simulink model "hcu_main_ADASwEPS"  (Simulink 8.2)
settings: Solver=FixedStepDiscrete  StartTime=0.0  StopTime=inf  FixedStep=0.001  RelTol=1e-3
PostLoadFcn:
  | , if any(exist('dsrtsu_mdlpostloadfcn', 'file') == [2, 3, 6]), try dsrtsu_mdlpostloadfcn('Execute', bdroot); catch fprintf('Error in PostLoadFcn (dsrtsu_mdlpostloadfcn) for model "%s":\n %s\n', bdroot, lasterr); end, end,
values from neighbouring files (symbols this model uses):
  C_TASK_1MS_S = (	C_TICK_TIME_S       )    [hcu_local_hdr.m]    (also in temp_ovrd_values.m = double(	0.001                  ))
  C_TICK_TIME_S = single(	0.005	    	)    [hcu_local_hdr.m]
  ENUM_EPSLFCSTATUS_ACTIVE = uint8(  2  )    [hcu_local_hdr.m]
  ENUM_EPSLFCSTATUS_TRANSITION = uint8(  3  )    [hcu_local_hdr.m]
  ENUM_EPSLKASTATUS_ACTIVE = uint8(  2  )    [hcu_local_hdr.m]
  ENUM_EPSMODEREQ_ANGLE = uint8(  1  )    [hcu_local_hdr.m]
  ENUM_EPSMODEREQ_INTERNAL = uint8(  0  )    [hcu_local_hdr.m]
  ENUM_EPSMODEREQ_TORQUE = uint8(  2  )    [hcu_local_hdr.m]
  ENUM_GEARPOSN_1ST = uint8(  1  )    [hcu_local_hdr.m]
  ENUM_GEARPOSN_2ND = uint8(  2  )    [hcu_local_hdr.m]
  ENUM_GEARPOSN_3RD = uint8(  3  )    [hcu_local_hdr.m]
  ENUM_GEARPOSN_4TH = uint8(  4  )    [hcu_local_hdr.m]
  ENUM_GEARPOSN_5TH = uint8(  5  )    [hcu_local_hdr.m]
  ENUM_GEARPOSN_6TH = uint8(  6  )    [hcu_local_hdr.m]
  ENUM_GEARPOSN_R = uint8(  7  )    [hcu_local_hdr.m]
  FALSE = boolean( 0 )    [hcu_local_hdr.m]
  TRUE = boolean( 1 )    [hcu_local_hdr.m]
undefined symbols (not defined in the file or in its folder): AISP_EPSCurrent_pct, AISP_TqASensorDelta_pct, AISP_TqBSensorDelta_pct, dHAL_IN, hal, INVALID_ABS1_TIMEOUT, INVALID_ABS2_TIMEOUT, INVALID_ABS3_TIMEOUT, INVALID_ABS4_TIMEOUT, INVALID_AC1_TIMEOUT, INVALID_ADASTORQ_REQ, INVALID_BCM1_TIMEOUT, INVALID_BCM2_TIMEOUT, INVALID_BOOSTER_VAC, INVALID_CSW1_TIMEOUT, INVALID_CUR_VEHDECE, INVALID_CURBRAKEDECE_REQ, INVALID_CURSTEERANG_REQ, INVALID_CURSTEERTQ_REQ, INVALID_ECM1_TIMEOUT, INVALID_ECM2_TIMEOUT, INVALID_ECM3_TIMEOUT, INVALID_ECM9_TIMEOUT, INVALID_ENG_TORQUE_FRICTIONAL, INVALID_ENG_TORQUE_INDICATED, INVALID_ENG_TORQUE_INDICATEDCOR, INVALID_ENG_TQ_MAX, INVALID_ENG_TQ_MIN, INVALID_EPAS2_TIMEOUT, INVALID_EPAS3_TIMEOUT, INVALID_EPB1_TIMEOUT, INVALID_EPS_BATTVOLT, INVALID_ESC_BATTVOLT, INVALID_GRADE, INVALID_HCU3_TIMEOUT, INVALID_HCU4_TIMEOUT, INVALID_HMI1_TIMEOUT, INVALID_HMI2_TIMEOUT, INVALID_LAT_ACC, INVALID_LONG_ACC, INVALID_MC_PRESSURE, INVALID_METER1_TIMEOUT, INVALID_METER3_TIMEOUT, INVALID_METER_VEHSPD, INVALID_ODO_METER, INVALID_OUTSIDE_TEMP, INVALID_PARKBRAKEBIND_STAT, INVALID_PEDALTQ_REQ, INVALID_SAS1_TIMEOUT, INVALID_SAS_ANGLE, INVALID_SHIFTER_POSN, INVALID_TCM1_TIMEOUT, INVALID_TCM2_TIMEOUT, INVALID_VCU1_TIMEOUT, INVALID_VCU2_TIMEOUT, INVALID_VEH_CRASH, INVALID_VEH_SPD, INVALID_WHEEL_SPD, INVALID_YAW_RATE, KHAL_MssgIdObj1_num ... (+8)
libraries: simulink x147, hcu_lib x38, rti1401lib_dio_type3 x4, rtimmsu_dsrtlib x3, app x1, rtiethernetudplib x1, rti1401lib_adc_type4 x1, rti1401lib_dac_type3 x1, inp x1, lidr x1, outp x1
(part 12 of 15)

== system hcu_main_ADASwEPS/dHAL_IN/HAL_IN_HMI/BO__1347_HMI1__8_HMI ==
  CAN1_Rx : Inport
  Bus Selector : BusSelector  OutputSignals=HMI1.ACCCancel,HMI1.ACCOn,HMI1.ACCRes_SpdInc,HMI1.ACCSet_SpdDec,HMI1.ACCSpeedDec,HMI1.ACCSpeedInc,HMI1.ACCTimeGapDec,HMI1.ACCTimeGapInc,HMI1.AEBEnable,HMI1.CSCEnable,HMI1.FCWEnable,HMI1.IGSAOn,HMI1.IGSARes_SpdInc,HMI1.IGSASet_SpdDec,HMI1.IGSASwitchMode,HMI1.LCSEnable,HMI1.LFC_PilotCancel,HMI1.LFC_PilotOn,HMI1.LKAEnable,HMI1.MAPAEnable,HMI1.FCWWarningMode,HMI1.DefMaxACCSetSpeed
  ACCCancel : Outport
  ACCOn : Outport  Port=2
  ACCRes_SpdInc : Outport  Port=3
  ACCSet_SpdDec : Outport  Port=4
  ACCSpeedDec : Outport  Port=5
  ACCSpeedInc : Outport  Port=6
  ACCTimeGapDec : Outport  Port=7
  ACCTimeGapInc : Outport  Port=8
  AEBEnable : Outport  Port=9
  CSCEnable : Outport  Port=10
  FCWEnable : Outport  Port=11
  IGSAOn : Outport  Port=12
  IGSARes_SpdInc : Outport  Port=13
  IGSASet_SpdDec : Outport  Port=14
  IGSASwitchMode : Outport  Port=15
  LCSEnable : Outport  Port=16
  LFC_PilotCancel : Outport  Port=17
  LFC_PilotOn : Outport  Port=18
  LKAEnable : Outport  Port=19
  MAPAEnable : Outport  Port=20
  FCWWarningMode : Outport  Port=21
  DefMaxACCSetSpeed : Outport  Port=22
  wires:
  [CAN1_Rx] -> Bus Selector/1
  CAN1_Rx/1 -> [CAN1_Rx]
  Bus Selector/1 -> ACCCancel/1  "<ACCCancel>"
  Bus Selector/2 -> ACCOn/1  "<ACCOn>"
  Bus Selector/3 -> ACCRes_SpdInc/1  "<ACCRes_SpdInc>"
  Bus Selector/4 -> ACCSet_SpdDec/1  "<ACCSet_SpdDec>"
  Bus Selector/5 -> ACCSpeedDec/1  "<ACCSpeedDec>"
  Bus Selector/6 -> ACCSpeedInc/1  "<ACCSpeedInc>"
  Bus Selector/7 -> ACCTimeGapDec/1  "<ACCTimeGapDec>"
  Bus Selector/8 -> ACCTimeGapInc/1  "<ACCTimeGapInc>"
  Bus Selector/9 -> AEBEnable/1  "<AEBEnable>"
  Bus Selector/10 -> CSCEnable/1  "<CSCEnable>"
  Bus Selector/11 -> FCWEnable/1  "<FCWEnable>"
  Bus Selector/16 -> LCSEnable/1  "<LCSEnable>"
  Bus Selector/17 -> LFC_PilotCancel/1  "<LFC_PilotCancel>"
  Bus Selector/18 -> LFC_PilotOn/1  "<LFC_PilotOn>"
  Bus Selector/19 -> LKAEnable/1  "<LKAEnable>"
  Bus Selector/20 -> MAPAEnable/1  "<MAPAEnable>"
  Bus Selector/12 -> IGSAOn/1  "<IGSAOn>"
  Bus Selector/13 -> IGSARes_SpdInc/1  "<IGSARes_SpdInc>"
  Bus Selector/14 -> IGSASet_SpdDec/1  "<IGSASet_SpdDec>"
  Bus Selector/15 -> IGSASwitchMode/1  "<IGSASwitchMode>"
  Bus Selector/21 -> FCWWarningMode/1  "<FCWWarningMode>"
  Bus Selector/22 -> DefMaxACCSetSpeed/1  "<DefMaxACCSetSpeed>"

== system hcu_main_ADASwEPS/dHAL_IN/HAL_IN_RadObjDecoder/RObj_Parser ==
  RObj_Status : Inport
  RObj_Frames1 : Inport  Port=2
  RObj_Frames2 : Inport  Port=3
  RObj_CollDetWarn : Inport  Port=4
  Ground : Ground
  Ground1 : Ground
  RObj_FramesParser : MATLAB Function  TreatAsAtomicUnit=on
  RObj_StatusParser : MATLAB Function  TreatAsAtomicUnit=on
  Terminator : Terminator
  VHAL_RadNofObjects_num : Outport
  VHAL_MeasCounter_num : Outport  Port=2
  VHAL_SensorRxInvalid_enum : Outport  Port=3
  VHAL_SensorSupplyVoltage_V : Outport  Port=4
  VHAL_SensorDefective_enum : Outport  Port=5
  VHAL_SensorMisaligned_enum : Outport  Port=6
  VHAL_SensorSwitchedOff_enum : Outport  Port=7
  VHAL_SensorExternalDisturbed_enum : Outport  Port=8
  VHAL_SensorOutputReduced_enum : Outport  Port=9
  VHAL_LatDistToborderLeft_m : Outport  Port=10
  VHAL_LatDistToborderRight_m : Outport  Port=11
  VHAL_RadObjRolCountVect40_num : Outport  Port=12
  VHAL_RadObjIDVect40_num : Outport  Port=13
  VHAL_RadObjXDisplVect40_m : Outport  Port=14
  VHAL_RadObjVrelXVect40_mps : Outport  Port=15
  VHAL_RadObjAccelXVect40_mps2 : Outport  Port=16
  VHAL_RadObjYDisplVect40_m : Outport  Port=17
  VHAL_RadObjDynPropVect40_enum : Outport  Port=18
  VHAL_RadObjPExistVect40_enum : Outport  Port=19
  VHAL_RadObjMeasStatVect40_enum : Outport  Port=20
  VHAL_RadObjWidthVect40_m : Outport  Port=21
  VHAL_RadObjLengthVect40_m : Outport  Port=22
  VHAL_RadObjRCSVect40_num : Outport  Port=23
  VHAL_RadObjVrelYVect40_mps : Outport  Port=24
  VHAL_RadObjProbVect40_num : Outport  Port=25
  VHAL_RadWarningLevel_enum : Outport  Port=26
  VHAL_RadWarningObjID_num : Outport  Port=27
  wires:
  RObj_Status/1 -> RObj_StatusParser/1(Status_Frame)
  RObj_FramesParser/1(Obj_RolCount) -> VHAL_RadObjRolCountVect40_num/1
  RObj_FramesParser/2(Obj_ID) -> VHAL_RadObjIDVect40_num/1
  RObj_FramesParser/3(Obj_LongDispl) -> VHAL_RadObjXDisplVect40_m/1
  RObj_FramesParser/4(Obj_VrelLong) -> VHAL_RadObjVrelXVect40_mps/1
  RObj_FramesParser/5(Obj_AccelLong) -> VHAL_RadObjAccelXVect40_mps2/1
  RObj_FramesParser/6(Obj_LatDispl) -> VHAL_RadObjYDisplVect40_m/1
  RObj_FramesParser/7(Obj_DynProp) -> VHAL_RadObjDynPropVect40_enum/1
  RObj_FramesParser/9(Obj_MeasStat) -> VHAL_RadObjMeasStatVect40_enum/1
  RObj_FramesParser/11(Obj_Length) -> VHAL_RadObjLengthVect40_m/1
  RObj_FramesParser/8(Obj_ProbOfExist) -> VHAL_RadObjPExistVect40_enum/1
  RObj_FramesParser/10(Obj_Width) -> VHAL_RadObjWidthVect40_m/1
  RObj_FramesParser/14(Obj_ObstacleProb) -> VHAL_RadObjProbVect40_num/1
  RObj_FramesParser/12(Obj_RCSValue) -> VHAL_RadObjRCSVect40_num/1
  RObj_FramesParser/13(Obj_LatSpeed) -> VHAL_RadObjVrelYVect40_mps/1
  RObj_Frames1/1 -> RObj_FramesParser/1(Frames1)
  RObj_Frames2/1 -> RObj_FramesParser/2(Frames2)
  RObj_StatusParser/1(N_of_Objects) -> VHAL_RadNofObjects_num/1
  RObj_StatusParser/6(SensorMisaligned) -> VHAL_SensorMisaligned_enum/1
  RObj_StatusParser/5(SensorDefective) -> VHAL_SensorDefective_enum/1
  RObj_StatusParser/8(SensorExternalDisturbed) -> VHAL_SensorExternalDisturbed_enum/1
  RObj_StatusParser/7(SensorSwitchedOff) -> VHAL_SensorSwitchedOff_enum/1
  RObj_StatusParser/9(SensorOutputReduced) -> VHAL_SensorOutputReduced_enum/1
  RObj_StatusParser/11(LatDistToborderRight) -> VHAL_LatDistToborderRight_m/1
  RObj_StatusParser/2(MeasCounter) -> VHAL_MeasCounter_num/1
  RObj_StatusParser/10(LatDistToborderLeft) -> VHAL_LatDistToborderLeft_m/1
  RObj_StatusParser/3(SensorRxInvalid) -> VHAL_SensorRxInvalid_enum/1
  RObj_StatusParser/4(SensorSupplyVoltage) -> VHAL_SensorSupplyVoltage_V/1
  RObj_CollDetWarn/1 -> Terminator/1
  Ground/1 -> VHAL_RadWarningLevel_enum/1
  Ground1/1 -> VHAL_RadWarningObjID_num/1

== system hcu_main_ADASwEPS/dHAL_IN/HAL_IN_RadObjDecoder/RObjectPackFrame ==
  CAN_Frames : Inport
  CaptureMessage1 : Inport  Port=2
  CaptureMessage2 : Inport  Port=3
  CaptureMessage3 : Inport  Port=4
  CaptureMessage4 : Inport  Port=5
  CaptureMessage5 : Inport  Port=6
  CaptureMessage6 : Inport  Port=7
  CaptureMessage7 : Inport  Port=8
  CaptureMessage8 : Inport  Port=9
  CaptureMessage9 : Inport  Port=10
  CaptureMessage10 : Inport  Port=11
  CaptureMessage11 : Inport  Port=12
  CaptureMessage12 : Inport  Port=13
  CaptureMessage13 : Inport  Port=14
  CaptureMessage14 : Inport  Port=15
  CaptureMessage15 : Inport  Port=16
  CaptureMessage16 : Inport  Port=17
  CaptureMessage17 : Inport  Port=18
  CaptureMessage18 : Inport  Port=19
  CaptureMessage19 : Inport  Port=20
  CaptureMessage20 : Inport  Port=21
  CaptureMessage21 : Inport  Port=22
  CaptureMessage22 : Inport  Port=23
  CaptureMessage23 : Inport  Port=24
  CaptureMessage24 : Inport  Port=25
  CaptureMessage25 : Inport  Port=26
  Bus Selector5 : BusSelector  OutputSignals=Status,ID,RAW_Byte_1,RAW_Byte_2,RAW_Byte_3,RAW_Byte_4,RAW_Byte_5,RAW_Byte_6,RAW_Byte_7,RAW_Byte_8
  Delay : Delay  DelayLength=1  InitialCondition=0
  For Iterator : ForIterator  IterationSource=external  IterationLimit=25
  Multiport Switch : MultiPortSwitch  Inputs=25
  RObjects_Decoder_v2 : Subsystem
  R_Objects_out : Outport  OutDataTypeStr=Bus: R_Objects
  wires:
  CaptureMessage1/1 -> Multiport Switch/2
  For Iterator/1 -> Multiport Switch/1
  CaptureMessage2/1 -> Multiport Switch/3
  CaptureMessage3/1 -> Multiport Switch/4
  CaptureMessage4/1 -> Multiport Switch/5
  CaptureMessage5/1 -> Multiport Switch/6
  CaptureMessage6/1 -> Multiport Switch/7
  CaptureMessage7/1 -> Multiport Switch/8
  CaptureMessage8/1 -> Multiport Switch/9
  CaptureMessage9/1 -> Multiport Switch/10
  CaptureMessage10/1 -> Multiport Switch/11
  CaptureMessage11/1 -> Multiport Switch/12
  CaptureMessage12/1 -> Multiport Switch/13
  CaptureMessage13/1 -> Multiport Switch/14
  CaptureMessage14/1 -> Multiport Switch/15
  CaptureMessage15/1 -> Multiport Switch/16
  CaptureMessage16/1 -> Multiport Switch/17
  CaptureMessage17/1 -> Multiport Switch/18
  CaptureMessage18/1 -> Multiport Switch/19
  CaptureMessage19/1 -> Multiport Switch/20
  CaptureMessage20/1 -> Multiport Switch/21
  CaptureMessage21/1 -> Multiport Switch/22
  CaptureMessage22/1 -> Multiport Switch/23
  CaptureMessage23/1 -> Multiport Switch/24
  CaptureMessage24/1 -> Multiport Switch/25
  CaptureMessage25/1 -> Multiport Switch/26
  RObjects_Decoder_v2/1(R_Objects_out) -> Delay/1, R_Objects_out/1
  Multiport Switch/1 -> Bus Selector5/1
  Bus Selector5/2 -> RObjects_Decoder_v2/2(ID)  "<ID>"
  Bus Selector5/4 -> RObjects_Decoder_v2/4(Byte2)  "<RAW_Byte_2>"
  Bus Selector5/3 -> RObjects_Decoder_v2/3(Byte1)  "<RAW_Byte_1>"
  Bus Selector5/10 -> RObjects_Decoder_v2/10(Byte8)  "<RAW_Byte_8>"
  Bus Selector5/1 -> RObjects_Decoder_v2/1(Status)  "<Status>"
  Bus Selector5/8 -> RObjects_Decoder_v2/8(Byte6)  "<RAW_Byte_6>"
  Bus Selector5/9 -> RObjects_Decoder_v2/9(Byte7)  "<RAW_Byte_7>"
  Bus Selector5/5 -> RObjects_Decoder_v2/5(Byte3)  "<RAW_Byte_3>"
  Bus Selector5/7 -> RObjects_Decoder_v2/7(Byte5)  "<RAW_Byte_5>"
  Bus Selector5/6 -> RObjects_Decoder_v2/6(Byte4)  "<RAW_Byte_4>"
  Delay/1 -> RObjects_Decoder_v2/11(R_Objects_in)
  CAN_Frames/1 -> For Iterator/1

== system hcu_main_ADASwEPS/dHAL_IN/HAL_IN_VCU/ADASTqReq_cvt ==
  value : Inport
  Add : Sum  Inputs=+-
  Data Type Conversion : DataTypeConversion  OutDataTypeStr=uint32  RndMeth=Nearest
  Divide : Product  Inputs=*/
  gain : Constant  Value=single(gain)  OutDataTypeStr=single
  offset : Constant  Value=single(offset)  OutDataTypeStr=single
  raw32 : Outport
  wires:
  Data Type Conversion/1 -> raw32/1
  gain/1 -> Divide/2
  Add/1 -> Divide/1
  Divide/1 -> Data Type Conversion/1
  offset/1 -> Add/2
  value/1 -> Add/1

== system hcu_main_ADASwEPS/dHAL_IN/HAL_IN_VCU/BO__1344_HMI2__8_VCU ==
  CAN1_Rx : Inport
  Bus Selector : BusSelector  OutputSignals=HMI2.ACCOn_VCU,HMI2.ACCRes_SpdInc_VCU,HMI2.ACCSet_SpdDec_VCU,HMI2.ACCTimeGapInc_VCU,HMI2.ACCTimeGapDec_VCU,HMI2.LFCOn_VCU,HMI2.MSAOn_VCU
  ACCOn_VCU : Outport
  ACCRes_SpdInc_VCU : Outport  Port=2
  ACCSet_SpdDec_VCU : Outport  Port=3
  ACCTimeGapInc_VCU : Outport  Port=4
  ACCTimeGapDec_VCU : Outport  Port=5
  LFCOn_VCU : Outport  Port=6
  MSAOn_VCU : Outport  Port=7
  wires:
  CAN1_Rx/1 -> [CAN1_Rx]
  [CAN1_Rx] -> Bus Selector/1
  Bus Selector/1 -> ACCOn_VCU/1  "<ACCOn_VCU>"
  Bus Selector/2 -> ACCRes_SpdInc_VCU/1  "<ACCRes_SpdInc_VCU>"
  Bus Selector/3 -> ACCSet_SpdDec_VCU/1  "<ACCSet_SpdDec_VCU>"
  Bus Selector/4 -> ACCTimeGapInc_VCU/1  "<ACCTimeGapInc_VCU>"
  Bus Selector/5 -> ACCTimeGapDec_VCU/1  "<ACCTimeGapDec_VCU>"
  Bus Selector/6 -> LFCOn_VCU/1  "<LFCOn_VCU>"
  Bus Selector/7 -> MSAOn_VCU/1  "<MSAOn_VCU>"

== system hcu_main_ADASwEPS/dHAL_IN/HAL_IN_VCU/BO__1360_VCU1__8_VCU ==
  CAN1_Rx : Inport
  Bus Selector : BusSelector  OutputSignals=VCU1.CurBrakeDecReq,VCU1.CurBrakeDecReq_A,VCU1.ADASTqReq,VCU1.ADASTqReq_A,VCU1.CurVehDec,VCU1.DecContMan,VCU1.DriverBrakeSw,VCU1.DriverBrakeSw_V,VCU1.ExtTqAvail,VCU1.ECMTqSrc,VCU1.ESCBrkSta,VCU1.ESCExtBrkAvail,VCU1.VCUFault,VCU1.VCUBattVolt,VCU1.VCU1_Checksum,VCU1.VCU1_LifeCount
  ChecksumCalculation : Subsystem  TreatAsAtomicUnit=on
  CurBrakeDecReq : Outport
  CurBrakeDecReq_A : Outport  Port=2
  ADASTqReq : Outport  Port=3
  ADASTqReq_A : Outport  Port=4
  CurVehDec : Outport  Port=5
  DecContMan : Outport  Port=6
  DriverBrakeSw : Outport  Port=7
  DriverBrakeSw_V : Outport  Port=8
  ExtTqAvail : Outport  Port=9
  ECMTqSrc : Outport  Port=10
  ESCBrkSta : Outport  Port=11
  ESCExtBrkAvail : Outport  Port=12
  VCUFault : Outport  Port=13
  VCUBattVolt : Outport  Port=14
  VCU1_LifeCount : Outport  Port=15
  VCU1_Checksum : Outport  Port=16
  Message_Checksum : Outport  Port=17
  wires:
  [CAN1_Rx] -> Bus Selector/1
  CAN1_Rx/1 -> [CAN1_Rx]
  Bus Selector/1 -> CurBrakeDecReq/1  "<CurBrakeDecReq>"
  Bus Selector/5 -> CurVehDec/1  "<CurVehDec>"
  Bus Selector/6 -> DecContMan/1  "<DecContMan>"
  Bus Selector/7 -> DriverBrakeSw/1  "<DriverBrakeSw>"
  Bus Selector/2 -> CurBrakeDecReq_A/1  "<CurBrakeDecReq_A>"
  [CAN1_Rx] -> ChecksumCalculation/1(CAN1_Rx)
  ChecksumCalculation/1(Message_Checksum) -> Message_Checksum/1
  Bus Selector/3 -> ADASTqReq/1  "<ADASTqReq>"
  Bus Selector/4 -> ADASTqReq_A/1  "<ADASTqReq_A>"
  Bus Selector/8 -> DriverBrakeSw_V/1  "<DriverBrakeSw_V>"
  Bus Selector/9 -> ExtTqAvail/1  "<ExtTqAvail>"
  Bus Selector/10 -> ECMTqSrc/1  "<ECMTqSrc>"
  Bus Selector/11 -> ESCBrkSta/1  "<ESCBrkSta>"
  Bus Selector/12 -> ESCExtBrkAvail/1  "<ESCExtBrkAvail>"
  Bus Selector/13 -> VCUFault/1  "<VCUFault>"
  Bus Selector/14 -> VCUBattVolt/1  "<VCUBattVolt>"
  Bus Selector/15 -> VCU1_Checksum/1  "<VCU1_Checksum>"
  Bus Selector/16 -> VCU1_LifeCount/1  "<VCU1_LifeCount>"

== system hcu_main_ADASwEPS/dHAL_IN/HAL_IN_VCU/BO__1361_VCU2__8_VCU ==
  CAN1_Rx : Inport
  Bus Selector : BusSelector  OutputSignals=VCU2.VCU_AccelPedalPosn,VCU2.VCU_AccelPedalPosn_V,VCU2.PedalTqReq,VCU2.ADAS_GearPosnReq_ALLOW,VCU2.MSAStatus,VCU2.VCU2_LifeCount,VCU2.VCU2_Checksum
  ChecksumCalculation : Subsystem  TreatAsAtomicUnit=on
  VCU_AccelPedalPosn : Outport
  VCU_AccelPedalPosn_V : Outport  Port=2
  PedalTqReq : Outport  Port=3
  ADAS_GearPosnReq_ALLOW : Outport  Port=4
  MSAStatus : Outport  Port=5
  VCU2_LifeCount : Outport  Port=6
  VCU2_Checksum : Outport  Port=7
  Message_Checksum : Outport  Port=8
  wires:
  CAN1_Rx/1 -> [CAN1_Rx]
  [CAN1_Rx] -> Bus Selector/1
  [CAN1_Rx] -> ChecksumCalculation/1(CAN1_Rx)
  ChecksumCalculation/1(Message_Checksum) -> Message_Checksum/1
  Bus Selector/1 -> VCU_AccelPedalPosn/1  "<VCU_AccelPedalPosn>"
  Bus Selector/2 -> VCU_AccelPedalPosn_V/1  "<VCU_AccelPedalPosn_V>"
  Bus Selector/7 -> VCU2_Checksum/1  "<VCU2_Checksum>"
  Bus Selector/6 -> VCU2_LifeCount/1  "<VCU2_LifeCount>"
  Bus Selector/3 -> PedalTqReq/1  "<PedalTqReq>"
  Bus Selector/4 -> ADAS_GearPosnReq_ALLOW/1  "<ADAS_GearPosnReq_ALLOW>"
  Bus Selector/5 -> MSAStatus/1  "<MSAStatus>"

== system hcu_main_ADASwEPS/dHAL_IN/HAL_IN_VCU/BO__883_HCU3__8_VCU ==
  CAN1_Rx : Inport
  Bus Selector : BusSelector  OutputSignals=HCU3.HybridLimpHome,HCU3.HCU3RollCnt
  HybridLimpHome : Outport
  HCU3RollCnt : Outport  Port=2
  wires:
  CAN1_Rx/1 -> [CAN1_Rx]
  [CAN1_Rx] -> Bus Selector/1
  Bus Selector/2 -> HCU3RollCnt/1  "<HCU3RollCnt>"
  Bus Selector/1 -> HybridLimpHome/1  "<HybridLimpHome>"

== system hcu_main_ADASwEPS/dHAL_IN/HAL_IN_VCU/BO__899_HCU4__8_VCU ==
  CAN1_Rx : Inport
  Bus Selector : BusSelector  OutputSignals=HCU4.MILReq
  MILReq : Outport
  wires:
  [CAN1_Rx] -> Bus Selector/1
  CAN1_Rx/1 -> [CAN1_Rx]
  Bus Selector/1 -> MILReq/1  "<MILReq>"

== system hcu_main_ADASwEPS/dHAL_IN/HAL_IN_VCU/CurBrakeDecReq_cvt ==
  value : Inport
  Add : Sum  Inputs=+-
  Data Type Conversion : DataTypeConversion  OutDataTypeStr=uint32  RndMeth=Nearest
  Divide : Product  Inputs=*/
  gain : Constant  Value=single(gain)  OutDataTypeStr=single
  offset : Constant  Value=single(offset)  OutDataTypeStr=single
  raw32 : Outport
  wires:
  value/1 -> Add/1
  offset/1 -> Add/2
  Divide/1 -> Data Type Conversion/1
  Add/1 -> Divide/1
  gain/1 -> Divide/2
  Data Type Conversion/1 -> raw32/1

== system hcu_main_ADASwEPS/dHAL_IN/HAL_IN_VCU/CurVehDec_cvt ==
  value : Inport
  Add : Sum  Inputs=+-
  Data Type Conversion : DataTypeConversion  OutDataTypeStr=uint32  RndMeth=Nearest
  Divide : Product  Inputs=*/
  gain : Constant  Value=single(gain)  OutDataTypeStr=single
  offset : Constant  Value=single(offset)  OutDataTypeStr=single
  raw32 : Outport
  wires:
  value/1 -> Add/1
  offset/1 -> Add/2
  Divide/1 -> Data Type Conversion/1
  Add/1 -> Divide/1
  gain/1 -> Divide/2
  Data Type Conversion/1 -> raw32/1

== system hcu_main_ADASwEPS/dHAL_IN/HAL_IN_VCU/PedalTqReq_cvt ==
  value : Inport
  Add : Sum  Inputs=+-
  Data Type Conversion : DataTypeConversion  OutDataTypeStr=uint32  RndMeth=Nearest
  Divide : Product  Inputs=*/
  gain : Constant  Value=single(gain)  OutDataTypeStr=single
  offset : Constant  Value=single(offset)  OutDataTypeStr=single
  raw32 : Outport
  wires:
  Data Type Conversion/1 -> raw32/1
  gain/1 -> Divide/2
  Add/1 -> Divide/1
  Divide/1 -> Data Type Conversion/1
  offset/1 -> Add/2
  value/1 -> Add/1

== system hcu_main_ADASwEPS/dHAL_IN/HAL_IN_VCU/VCUBattVolt_cvt ==
  value : Inport
  Add : Sum  Inputs=+-
  Data Type Conversion : DataTypeConversion  OutDataTypeStr=uint32  RndMeth=Nearest
  Divide : Product  Inputs=*/
  gain : Constant  Value=single(gain)  OutDataTypeStr=single
  offset : Constant  Value=single(offset)  OutDataTypeStr=single
  raw32 : Outport
  wires:
  Data Type Conversion/1 -> raw32/1
  gain/1 -> Divide/2
  Add/1 -> Divide/1
  Divide/1 -> Data Type Conversion/1
  offset/1 -> Add/2
  value/1 -> Add/1

== system hcu_main_ADASwEPS/dHAL_IN/dHAL_IN_ABS/BO_864_ABS2_8_ABS ==
  CAN1_Rx : Inport
  Bus Selector : BusSelector  OutputSignals=ABS2.ABS_Active,ABS2.ABS_Failed,ABS2.BrkSw_Sta,ABS2.BrkSw_V,ABS2.EBD_Failed,ABS2.ESC_Active,ABS2.ESC_Failed,ABS2.HSA_Active,ABS2.HSA_Failed,ABS2.TCS_Active,ABS2.TCS_Enabled,ABS2.TCS_Failed,ABS2.VehSpeed,ABS2.VehSpeed_Checksum,ABS2.VehSpeed_LifeCount
  ChecksumCalculation : Subsystem  TreatAsAtomicUnit=on
  ABS_Active : Outport
  ABS_Failed : Outport  Port=2
  BrkSw_Sta : Outport  Port=3
  BrkSw_V : Outport  Port=4
  EBD_Failed : Outport  Port=5
  ESC_Active : Outport  Port=6
  ESC_Failed : Outport  Port=7
  HSA_Active : Outport  Port=8
  HSA_Failed : Outport  Port=9
  TCS_Active : Outport  Port=10
  TCS_Enabled : Outport  Port=11
  TCS_Failed : Outport  Port=12
  VehSpeed : Outport  Port=13
  VehSpeed_LifeCount : Outport  Port=14
  VehSpeed_Checksum : Outport  Port=15
  Message_Checksum : Outport  Port=16
  wires:
  [CAN1_Rx] -> Bus Selector/1
  CAN1_Rx/1 -> [CAN1_Rx]
  Bus Selector/1 -> ABS_Active/1  "<ABS_Active>"
  Bus Selector/2 -> ABS_Failed/1  "<ABS_Failed>"
  Bus Selector/3 -> BrkSw_Sta/1  "<BrkSw_Sta>"
  Bus Selector/4 -> BrkSw_V/1  "<BrkSw_V>"
  Bus Selector/5 -> EBD_Failed/1  "<EBD_Failed>"
  Bus Selector/6 -> ESC_Active/1  "<ESC_Active>"
  Bus Selector/7 -> ESC_Failed/1  "<ESC_Failed>"
  Bus Selector/8 -> HSA_Active/1  "<HSA_Active>"
  Bus Selector/9 -> HSA_Failed/1  "<HSA_Failed>"
  Bus Selector/10 -> TCS_Active/1  "<TCS_Active>"
  Bus Selector/11 -> TCS_Enabled/1  "<TCS_Enabled>"
  Bus Selector/12 -> TCS_Failed/1  "<TCS_Failed>"
  Bus Selector/13 -> VehSpeed/1  "<VehSpeed>"
  Bus Selector/14 -> VehSpeed_Checksum/1  "<VehSpeed_Checksum>"
  Bus Selector/15 -> VehSpeed_LifeCount/1  "<VehSpeed_LifeCount>"
  [CAN1_Rx] -> ChecksumCalculation/1(CAN1_Rx)
  ChecksumCalculation/1(Message_Checksum) -> Message_Checksum/1

== system hcu_main_ADASwEPS/dHAL_IN/dHAL_IN_ABS/BO__848_ABS1__8_ABS ==
  CAN1_Rx : Inport
  Bus Selector : BusSelector  OutputSignals=ABS1.BoosterVac,ABS1.BoosterVac_Sta,ABS1.BoosterVac_V,ABS1.GRADE,ABS1.GRADE_V,ABS1.TCSRollCnt
  BoosterVac : Outport
  BoosterVac_V : Outport  Port=2
  BoosterVac_Sta : Outport  Port=3
  GRADE : Outport  Port=4
  GRADE_V : Outport  Port=5
  TCSRollCnt : Outport  Port=6
  wires:
  [CAN1_Rx] -> Bus Selector/1
  CAN1_Rx/1 -> [CAN1_Rx]
  Bus Selector/1 -> BoosterVac/1  "<BoosterVac>"
  Bus Selector/2 -> BoosterVac_Sta/1  "<BoosterVac_Sta>"
  Bus Selector/3 -> BoosterVac_V/1  "<BoosterVac_V>"
  Bus Selector/4 -> GRADE/1  "<GRADE>"
  Bus Selector/5 -> GRADE_V/1  "<GRADE_V>"
  Bus Selector/6 -> TCSRollCnt/1  "<TCSRollCnt>"

== system hcu_main_ADASwEPS/dHAL_IN/dHAL_IN_ABS/BO__880_ABS3__8_ABS ==
  CAN1_Rx : Inport
  Bus Selector : BusSelector  OutputSignals=ABS3.LF_RawWhlSpeed,ABS3.LF_RawWhlSpeed_V,ABS3.LR_RawWhlSpeed,ABS3.LR_RawWhlSpeed_V,ABS3.RF_RawWhlSpeed,ABS3.RF_RawWhlSpeed_V,ABS3.RR_RawWhlSpeed,ABS3.RR_RawWhlSpeed_V
  LF_RawWhlSpeed : Outport
  LF_RawWhlSpeed_V : Outport  Port=2
  LR_RawWhlSpeed : Outport  Port=3
  LR_RawWhlSpeed_V : Outport  Port=4
  RF_RawWhlSpeed : Outport  Port=5
  RF_RawWhlSpeed_V : Outport  Port=6
  RR_RawWhlSpeed : Outport  Port=7
  RR_RawWhlSpeed_V : Outport  Port=8
  wires:
  CAN1_Rx/1 -> [CAN1_Rx]
  [CAN1_Rx] -> Bus Selector/1
  Bus Selector/1 -> LF_RawWhlSpeed/1  "<LF_RawWhlSpeed>"
  Bus Selector/2 -> LF_RawWhlSpeed_V/1  "<LF_RawWhlSpeed_V>"
  Bus Selector/3 -> LR_RawWhlSpeed/1  "<LR_RawWhlSpeed>"
  Bus Selector/4 -> LR_RawWhlSpeed_V/1  "<LR_RawWhlSpeed_V>"
  Bus Selector/5 -> RF_RawWhlSpeed/1  "<RF_RawWhlSpeed>"
  Bus Selector/6 -> RF_RawWhlSpeed_V/1  "<RF_RawWhlSpeed_V>"
  Bus Selector/7 -> RR_RawWhlSpeed/1  "<RR_RawWhlSpeed>"
  Bus Selector/8 -> RR_RawWhlSpeed_V/1  "<RR_RawWhlSpeed_V>"

== system hcu_main_ADASwEPS/dHAL_IN/dHAL_IN_ABS/BO__896_ABS4__8_ABS ==
  CAN1_Rx : Inport
  Bus Selector : BusSelector  OutputSignals=ABS4.LatAccel,ABS4.LatAccel_V,ABS4.LongAccel,ABS4.LongAccel_V,ABS4.MCPressure,ABS4.MCPressure_V,ABS4.YawRate,ABS4.YawRate_V
  LatAccel : Outport
  LatAccel_V : Outport  Port=2
  LongAccel : Outport  Port=3
  LongAccel_V : Outport  Port=4
  MCPressure : Outport  Port=5
  MCPressure_V : Outport  Port=6
  YawRate : Outport  Port=7
  YawRate_V : Outport  Port=8
  wires:
  CAN1_Rx/1 -> [CAN1_Rx]
  [CAN1_Rx] -> Bus Selector/1
  Bus Selector/1 -> LatAccel/1  "<LatAccel>"
  Bus Selector/2 -> LatAccel_V/1  "<LatAccel_V>"
  Bus Selector/3 -> LongAccel/1  "<LongAccel>"
  Bus Selector/4 -> LongAccel_V/1  "<LongAccel_V>"
  Bus Selector/5 -> MCPressure/1  "<MCPressure>"
  Bus Selector/6 -> MCPressure_V/1  "<MCPressure_V>"
  Bus Selector/7 -> YawRate/1  "<YawRate>"
  Bus Selector/8 -> YawRate_V/1  "<YawRate_V>"

== system hcu_main_ADASwEPS/dHAL_IN/dHAL_IN_ABS/BoosterVac_cvt ==
  value : Inport
  Add : Sum  Inputs=+-
  Data Type Conversion : DataTypeConversion  OutDataTypeStr=uint32  RndMeth=Nearest
  Divide : Product  Inputs=*/
  gain : Constant  Value=single(gain)  OutDataTypeStr=single
  offset : Constant  Value=single(offset)  OutDataTypeStr=single
  raw32 : Outport
  wires:
  Data Type Conversion/1 -> raw32/1
  gain/1 -> Divide/2
  Add/1 -> Divide/1
  Divide/1 -> Data Type Conversion/1
  offset/1 -> Add/2
  value/1 -> Add/1

== system hcu_main_ADASwEPS/dHAL_IN/dHAL_IN_ABS/GRADE_cvt ==
  value : Inport
  Add : Sum  Inputs=+-
  Data Type Conversion : DataTypeConversion  OutDataTypeStr=uint32  RndMeth=Nearest
  Divide : Product  Inputs=*/
  gain : Constant  Value=single(gain)  OutDataTypeStr=single
  offset : Constant  Value=single(offset)  OutDataTypeStr=single
  raw32 : Outport
  wires:
  value/1 -> Add/1
  offset/1 -> Add/2
  Divide/1 -> Data Type Conversion/1
  Add/1 -> Divide/1
  gain/1 -> Divide/2
  Data Type Conversion/1 -> raw32/1

== system hcu_main_ADASwEPS/dHAL_IN/dHAL_IN_ABS/LF_RawWhlSpeed_cvt ==
  value : Inport
  Add : Sum  Inputs=+-
  Data Type Conversion : DataTypeConversion  OutDataTypeStr=uint32  RndMeth=Nearest
  Divide : Product  Inputs=*/
  gain : Constant  Value=single(gain)  OutDataTypeStr=single
  offset : Constant  Value=single(offset)  OutDataTypeStr=single
  raw32 : Outport
  wires:
  Data Type Conversion/1 -> raw32/1
  gain/1 -> Divide/2
  Add/1 -> Divide/1
  Divide/1 -> Data Type Conversion/1
  offset/1 -> Add/2
  value/1 -> Add/1

== system hcu_main_ADASwEPS/dHAL_IN/dHAL_IN_ABS/LR_RawWhlSpeed_cvt ==
  value : Inport
  Add : Sum  Inputs=+-
  Data Type Conversion : DataTypeConversion  OutDataTypeStr=uint32  RndMeth=Nearest
  Divide : Product  Inputs=*/
  gain : Constant  Value=single(gain)  OutDataTypeStr=single
  offset : Constant  Value=single(offset)  OutDataTypeStr=single
  raw32 : Outport
  wires:
  value/1 -> Add/1
  offset/1 -> Add/2
  Divide/1 -> Data Type Conversion/1
  Add/1 -> Divide/1
  gain/1 -> Divide/2
  Data Type Conversion/1 -> raw32/1

== system hcu_main_ADASwEPS/dHAL_IN/dHAL_IN_ABS/LatAccel_cvt ==
  value : Inport
  Add : Sum  Inputs=+-
  Data Type Conversion : DataTypeConversion  OutDataTypeStr=uint32  RndMeth=Nearest
  Divide : Product  Inputs=*/
  gain : Constant  Value=single(gain)  OutDataTypeStr=single
  offset : Constant  Value=single(offset)  OutDataTypeStr=single
  raw32 : Outport
  wires:
  Data Type Conversion/1 -> raw32/1
  gain/1 -> Divide/2
  Add/1 -> Divide/1
  Divide/1 -> Data Type Conversion/1
  offset/1 -> Add/2
  value/1 -> Add/1

== system hcu_main_ADASwEPS/dHAL_IN/dHAL_IN_ABS/LongAccel_cvt ==
  value : Inport
  Add : Sum  Inputs=+-
  Data Type Conversion : DataTypeConversion  OutDataTypeStr=uint32  RndMeth=Nearest
  Divide : Product  Inputs=*/
  gain : Constant  Value=single(gain)  OutDataTypeStr=single
  offset : Constant  Value=single(offset)  OutDataTypeStr=single
  raw32 : Outport
  wires:
  value/1 -> Add/1
  offset/1 -> Add/2
  Divide/1 -> Data Type Conversion/1
  Add/1 -> Divide/1
  gain/1 -> Divide/2
  Data Type Conversion/1 -> raw32/1

== system hcu_main_ADASwEPS/dHAL_IN/dHAL_IN_ABS/MCPressure_cvt ==
  value : Inport
  Add : Sum  Inputs=+-
  Data Type Conversion : DataTypeConversion  OutDataTypeStr=uint32  RndMeth=Nearest
  Divide : Product  Inputs=*/
  gain : Constant  Value=single(gain)  OutDataTypeStr=single
  offset : Constant  Value=single(offset)  OutDataTypeStr=single
  raw32 : Outport
  wires:
  Data Type Conversion/1 -> raw32/1
  gain/1 -> Divide/2
  Add/1 -> Divide/1
  Divide/1 -> Data Type Conversion/1
  offset/1 -> Add/2
  value/1 -> Add/1

== system hcu_main_ADASwEPS/dHAL_IN/dHAL_IN_ABS/RF_RawWhlSpeed_cvt ==
  value : Inport
  Add : Sum  Inputs=+-
  Data Type Conversion : DataTypeConversion  OutDataTypeStr=uint32  RndMeth=Nearest
  Divide : Product  Inputs=*/
  gain : Constant  Value=single(gain)  OutDataTypeStr=single
  offset : Constant  Value=single(offset)  OutDataTypeStr=single
  raw32 : Outport
  wires:
  Data Type Conversion/1 -> raw32/1
  gain/1 -> Divide/2
  Add/1 -> Divide/1
  Divide/1 -> Data Type Conversion/1
  offset/1 -> Add/2
  value/1 -> Add/1

== system hcu_main_ADASwEPS/dHAL_IN/dHAL_IN_ABS/RR_RawWhlSpeed_cvt ==
  value : Inport
  Add : Sum  Inputs=+-
  Data Type Conversion : DataTypeConversion  OutDataTypeStr=uint32  RndMeth=Nearest
  Divide : Product  Inputs=*/
  gain : Constant  Value=single(gain)  OutDataTypeStr=single
  offset : Constant  Value=single(offset)  OutDataTypeStr=single
  raw32 : Outport
  wires:
  value/1 -> Add/1
  offset/1 -> Add/2
  Divide/1 -> Data Type Conversion/1
  Add/1 -> Divide/1
  gain/1 -> Divide/2
  Data Type Conversion/1 -> raw32/1

== system hcu_main_ADASwEPS/dHAL_IN/dHAL_IN_ABS/VehSpeed_cvt ==
  value : Inport
  Add : Sum  Inputs=+-
  Data Type Conversion : DataTypeConversion  OutDataTypeStr=uint32  RndMeth=Nearest
  Divide : Product  Inputs=*/
  gain : Constant  Value=single(gain)  OutDataTypeStr=single
  offset : Constant  Value=single(offset)  OutDataTypeStr=single
  raw32 : Outport
  wires:
  Data Type Conversion/1 -> raw32/1
  gain/1 -> Divide/2
  Add/1 -> Divide/1
  Divide/1 -> Data Type Conversion/1
  offset/1 -> Add/2
  value/1 -> Add/1

== system hcu_main_ADASwEPS/dHAL_IN/dHAL_IN_ABS/YawRate_cvt ==
  value : Inport
  Add : Sum  Inputs=+-
  Data Type Conversion : DataTypeConversion  OutDataTypeStr=uint32  RndMeth=Nearest
  Divide : Product  Inputs=*/
  gain : Constant  Value=single(gain)  OutDataTypeStr=single
  offset : Constant  Value=single(offset)  OutDataTypeStr=single
  raw32 : Outport
  wires:
  value/1 -> Add/1
  offset/1 -> Add/2
  Divide/1 -> Data Type Conversion/1
  Add/1 -> Divide/1
  gain/1 -> Divide/2
  Data Type Conversion/1 -> raw32/1

== system hcu_main_ADASwEPS/dHAL_IN/dHAL_IN_AC/BO__1120_AC1__8_AC ==
  CAN1_Rx : Inport
  Bus Selector : BusSelector  OutputSignals=AC1.Sta_Out_Temp
  Sta_Out_Temp : Outport
  wires:
  [CAN1_Rx] -> Bus Selector/1
  CAN1_Rx/1 -> [CAN1_Rx]
  Bus Selector/1 -> Sta_Out_Temp/1  "<Sta_Out_Temp>"

== system hcu_main_ADASwEPS/dHAL_IN/dHAL_IN_AC/Sta_Out_Temp_cvt ==
  value : Inport
  Add : Sum  Inputs=+-
  Data Type Conversion : DataTypeConversion  OutDataTypeStr=uint32  RndMeth=Nearest
  Divide : Product  Inputs=*/
  gain : Constant  Value=single(gain)  OutDataTypeStr=single
  offset : Constant  Value=single(offset)  OutDataTypeStr=single
  raw32 : Outport
  wires:
  value/1 -> Add/1
  offset/1 -> Add/2
  Divide/1 -> Data Type Conversion/1
  Add/1 -> Divide/1
  gain/1 -> Divide/2
  Data Type Conversion/1 -> raw32/1

== system hcu_main_ADASwEPS/dHAL_IN/dHAL_IN_BCM/BO__1008_BCM2__8_BCM ==
  CAN1_Rx : Inport
  Bus Selector : BusSelector  OutputSignals=BCM2.BCM_SRS_Crash_Info
  BCM_SRS_Crash_Info : Outport
  wires:
  [CAN1_Rx] -> Bus Selector/1
  CAN1_Rx/1 -> [CAN1_Rx]
  Bus Selector/1 -> BCM_SRS_Crash_Info/1  "<BCM_SRS_Crash_Info>"

== system hcu_main_ADASwEPS/dHAL_IN/dHAL_IN_BCM/BO__1056_BCM1__8_BCM ==
  CAN1_Rx : Inport
  Bus Selector : BusSelector  OutputSignals=BCM1.BCM_AllDrSw_Sta,BCM1.BCM_DDrSw_Sta,BCM1.BCM_Hazard_Sta,BCM1.BCM_Key_Sta,BCM1.BCM_LRDrSw_Sta,BCM1.BCM_LTurnLp_Sta,BCM1.BCM_PDrSw_Sta,BCM1.BCM_RRDrSw_Sta,BCM1.BCM_RTurnLp_Sta,BCM1.BCM_TGateSw_Sta
  BCM_AllDrSw_Sta : Outport
  BCM_DDrSw_Sta : Outport  Port=2
  BCM_Hazard_Sta : Outport  Port=3
  BCM_Key_Sta : Outport  Port=4
  BCM_LRDrSw_Sta : Outport  Port=5
  BCM_LTurnLp_Sta : Outport  Port=6
  BCM_PDrSw_Sta : Outport  Port=7
  BCM_RRDrSw_Sta : Outport  Port=8
  BCM_RTurnLp_Sta : Outport  Port=9
  BCM_TGateSw_Sta : Outport  Port=10
  wires:
  CAN1_Rx/1 -> [CAN1_Rx]
  [CAN1_Rx] -> Bus Selector/1
  Bus Selector/1 -> BCM_AllDrSw_Sta/1  "<BCM_AllDrSw_Sta>"
  Bus Selector/2 -> BCM_DDrSw_Sta/1  "<BCM_DDrSw_Sta>"
  Bus Selector/3 -> BCM_Hazard_Sta/1  "<BCM_Hazard_Sta>"
  Bus Selector/4 -> BCM_Key_Sta/1  "<BCM_Key_Sta>"
  Bus Selector/5 -> BCM_LRDrSw_Sta/1  "<BCM_LRDrSw_Sta>"
  Bus Selector/6 -> BCM_LTurnLp_Sta/1  "<BCM_LTurnLp_Sta>"
  Bus Selector/7 -> BCM_PDrSw_Sta/1  "<BCM_PDrSw_Sta>"
  Bus Selector/8 -> BCM_RRDrSw_Sta/1  "<BCM_RRDrSw_Sta>"
  Bus Selector/9 -> BCM_RTurnLp_Sta/1  "<BCM_RTurnLp_Sta>"
  Bus Selector/10 -> BCM_TGateSw_Sta/1  "<BCM_TGateSw_Sta>"

== system hcu_main_ADASwEPS/dHAL_IN/dHAL_IN_ECM/BO_790_ECM1_8_ECM ==
  CAN1_Rx : Inport
  Bus Selector : BusSelector  OutputSignals=ECM1.CAN_N,ECM1.CAN_TQFR,ECM1.CAN_TQI,ECM1.CAN_TQI_ACOR,ECM1.LV_CAN_N_ERR,ECM1.LV_CAN_SUB_TQI
  CAN_N : Outport
  CAN_TQFR : Outport  Port=2
  CAN_TQI : Outport  Port=3
  CAN_TQI_ACOR : Outport  Port=4
  LV_CAN_N_ERR : Outport  Port=5
  LV_CAN_SUB_TQI : Outport  Port=6
  wires:
  Bus Selector/1 -> CAN_N/1  "<CAN_N>"
  Bus Selector/2 -> CAN_TQFR/1  "<CAN_TQFR>"
  Bus Selector/3 -> CAN_TQI/1  "<CAN_TQI>"
  Bus Selector/4 -> CAN_TQI_ACOR/1  "<CAN_TQI_ACOR>"
  Bus Selector/5 -> LV_CAN_N_ERR/1  "<LV_CAN_N_ERR>"
  Bus Selector/6 -> LV_CAN_SUB_TQI/1  "<LV_CAN_SUB_TQI>"
  CAN1_Rx/1 -> [CAN1_Rx]
  [CAN1_Rx] -> Bus Selector/1

== system hcu_main_ADASwEPS/dHAL_IN/dHAL_IN_ECM/BO_809_ECM2_8_ECM ==
  CAN1_Rx : Inport
  Bus Selector : BusSelector  OutputSignals=ECM2.Eng_Hood_SW,ECM2.CAN_OBD_STAT_WU,ECM2.CAN_OBD_STAT_DR
  Eng_Hood_SW : Outport
  CAN_OBD_STAT_WU : Outport  Port=2
  CAN_OBD_STAT_DR : Outport  Port=3
  wires:
  CAN1_Rx/1 -> Bus Selector/1
  Bus Selector/2 -> CAN_OBD_STAT_WU/1  "<CAN_OBD_STAT_WU>"
  Bus Selector/1 -> Eng_Hood_SW/1  "<Eng_Hood_SW>"
  Bus Selector/3 -> CAN_OBD_STAT_DR/1  "<CAN_OBD_STAT_DR>"

== system hcu_main_ADASwEPS/dHAL_IN/dHAL_IN_ECM/BO_821_ECM3_8_ECM ==
  CAN1_Rx : Inport
  Bus Selector : BusSelector  OutputSignals=ECM3.CAN_PV_AV,ECM3.CAN_PV_EFC,ECM3.LV_CAN_ERRPAS,ECM3.LV_CAN_ERRPVS
  CAN_PV_AV : Outport
  CAN_PV_EFC : Outport  Port=2
  LV_CAN_ERRPAS : Outport  Port=3
  LV_CAN_ERRPVS : Outport  Port=4
  wires:
  CAN1_Rx/1 -> Bus Selector/1
  Bus Selector/1 -> CAN_PV_AV/1  "<CAN_PV_AV>"
  Bus Selector/2 -> CAN_PV_EFC/1  "<CAN_PV_EFC>"
  Bus Selector/3 -> LV_CAN_ERRPAS/1  "<LV_CAN_ERRPAS>"
  Bus Selector/4 -> LV_CAN_ERRPVS/1  "<LV_CAN_ERRPVS>"

== system hcu_main_ADASwEPS/dHAL_IN/dHAL_IN_ECM/BO_875_ECM9_8_ECM ==
  CAN1_Rx1 : Inport
  Bus Selector : BusSelector  OutputSignals=ECM9.ECM9RollCnt,ECM9.EMSHybridOpState,ECM9.EMSOpState,ECM9.EngTqMax,ECM9.EngTqMin
  ECM9RollCnt : Outport
  EMSHybridOpState : Outport  Port=2
  EMSOpState : Outport  Port=3
  EngTqMax : Outport  Port=4
  EngTqMin : Outport  Port=5
  wires:
  Bus Selector/1 -> ECM9RollCnt/1  "<ECM9RollCnt>"
  Bus Selector/2 -> EMSHybridOpState/1  "<EMSHybridOpState>"
  Bus Selector/3 -> EMSOpState/1  "<EMSOpState>"
  Bus Selector/4 -> EngTqMax/1  "<EngTqMax>"
  Bus Selector/5 -> EngTqMin/1  "<EngTqMin>"
  CAN1_Rx1/1 -> [CAN1_Rx]
  [CAN1_Rx] -> Bus Selector/1

== system hcu_main_ADASwEPS/dHAL_IN/dHAL_IN_ECM/CAN_TQFR_cvt ==
  value : Inport
  Add : Sum  Inputs=+-
  Data Type Conversion : DataTypeConversion  OutDataTypeStr=uint32  RndMeth=Nearest
  Divide : Product  Inputs=*/
  gain : Constant  Value=single(gain)  OutDataTypeStr=single
  offset : Constant  Value=single(offset)  OutDataTypeStr=single
  raw32 : Outport
  wires:
  Data Type Conversion/1 -> raw32/1
  gain/1 -> Divide/2
  Add/1 -> Divide/1
  Divide/1 -> Data Type Conversion/1
  offset/1 -> Add/2
  value/1 -> Add/1

== system hcu_main_ADASwEPS/dHAL_IN/dHAL_IN_ECM/CAN_TQI_ACOR_cvt ==
  value : Inport
  Add : Sum  Inputs=+-
  Data Type Conversion : DataTypeConversion  OutDataTypeStr=uint32  RndMeth=Nearest
  Divide : Product  Inputs=*/
  gain : Constant  Value=single(gain)  OutDataTypeStr=single
  offset : Constant  Value=single(offset)  OutDataTypeStr=single
  raw32 : Outport
  wires:
  Data Type Conversion/1 -> raw32/1
  gain/1 -> Divide/2
  Add/1 -> Divide/1
  Divide/1 -> Data Type Conversion/1
  offset/1 -> Add/2
  value/1 -> Add/1

== system hcu_main_ADASwEPS/dHAL_IN/dHAL_IN_ECM/CAN_TQI_cvt ==
  value : Inport
  Add : Sum  Inputs=+-
  Data Type Conversion : DataTypeConversion  OutDataTypeStr=uint32  RndMeth=Nearest
  Divide : Product  Inputs=*/
  gain : Constant  Value=single(gain)  OutDataTypeStr=single
  offset : Constant  Value=single(offset)  OutDataTypeStr=single
  raw32 : Outport
  wires:
  value/1 -> Add/1
  offset/1 -> Add/2
  Divide/1 -> Data Type Conversion/1
  Add/1 -> Divide/1
  gain/1 -> Divide/2
  Data Type Conversion/1 -> raw32/1

== system hcu_main_ADASwEPS/dHAL_IN/dHAL_IN_ECM/EngTqMax_cvt ==
  value : Inport
  Add : Sum  Inputs=+-
  Data Type Conversion : DataTypeConversion  OutDataTypeStr=uint32  RndMeth=Nearest
  Divide : Product  Inputs=*/
  gain : Constant  Value=single(gain)  OutDataTypeStr=single
  offset : Constant  Value=single(offset)  OutDataTypeStr=single
  raw32 : Outport
  wires:
  value/1 -> Add/1
  offset/1 -> Add/2
  Divide/1 -> Data Type Conversion/1
  Add/1 -> Divide/1
  gain/1 -> Divide/2
  Data Type Conversion/1 -> raw32/1

== system hcu_main_ADASwEPS/dHAL_IN/dHAL_IN_ECM/EngTqMin_cvt ==
  value : Inport
  Add : Sum  Inputs=+-
  Data Type Conversion : DataTypeConversion  OutDataTypeStr=uint32  RndMeth=Nearest
  Divide : Product  Inputs=*/
  gain : Constant  Value=single(gain)  OutDataTypeStr=single
  offset : Constant  Value=single(offset)  OutDataTypeStr=single
  raw32 : Outport
  wires:
  Data Type Conversion/1 -> raw32/1
  gain/1 -> Divide/2
  Add/1 -> Divide/1
  Divide/1 -> Data Type Conversion/1
  offset/1 -> Add/2
  value/1 -> Add/1

== system hcu_main_ADASwEPS/dHAL_IN/dHAL_IN_EPAS/BO__1365_EPAS3__8_EPAS ==
  CAN1_Rx : Inport
  Bus Selector : BusSelector  OutputSignals=EPAS3.CurStrAngReq,EPAS3.CurStrAngReq_A,EPAS3.CurStrTqReq,EPAS3.CurStrTqReq_A,EPAS3.EPSBattVolt,EPAS3.EPSLKAStatus,EPAS3.EPSLFCStatus,EPAS3.EPSADASAbReason,EPAS3.EPAS3_Checksum,EPAS3.EPAS3_LifeCount
  ChecksumCalculation : Subsystem  TreatAsAtomicUnit=on
  CurStrAngReq : Outport
  CurStrAngReq_A : Outport  Port=2
  CurStrTqReq : Outport  Port=3
  CurStrTqReq_A : Outport  Port=4
  EPAS3_LifeCount : Outport  Port=5
  EPSBattVolt : Outport  Port=6
  EPSLKAStatus : Outport  Port=7
  EPSADASAbReason : Outport  Port=8
  EPSLFCStatus : Outport  Port=9
  EPAS3_Checksum : Outport  Port=10
  Message_Checksum : Outport  Port=11
  wires:
  [CAN1_Rx] -> ChecksumCalculation/2(CAN1_Rx)
  CAN1_Rx/1 -> [CAN1_Rx]
  [CAN1_Rx] -> Bus Selector/1
  Bus Selector/1 -> CurStrAngReq/1  "<CurStrAngReq>"
  Bus Selector/3 -> CurStrTqReq/1  "<CurStrTqReq>"
  Bus Selector/9 -> EPAS3_Checksum/1  "<EPAS3_Checksum>"
  Bus Selector/10 -> ChecksumCalculation/1(EPAS3_LifeCount), EPAS3_LifeCount/1  "<EPAS3_LifeCount>"
  Bus Selector/5 -> EPSBattVolt/1  "<EPSBattVolt>"
  ChecksumCalculation/1(Message_Checksum) -> Message_Checksum/1
  Bus Selector/6 -> EPSLKAStatus/1  "<EPSLKAStatus>"
  Bus Selector/8 -> EPSADASAbReason/1  "<EPSADASAbReason>"
  Bus Selector/7 -> EPSLFCStatus/1  "<EPSLFCStatus>"
  Bus Selector/2 -> CurStrAngReq_A/1  "<CurStrAngReq_A>"
  Bus Selector/4 -> CurStrTqReq_A/1  "<CurStrTqReq_A>"

== system hcu_main_ADASwEPS/dHAL_IN/dHAL_IN_EPAS/BO__922_SAS1__8_EPAS ==
  CAN1_Rx : Inport
  Bus Selector : BusSelector  OutputSignals=SAS1.SAS_Angle,SAS1.SAS_CAL,SAS1.SAS_CheckSum,SAS1.SAS_OK,SAS1.SAS_MsgCount
  ChecksumCalculation : Subsystem  TreatAsAtomicUnit=on
  SAS_Angle : Outport
  SAS_CAL : Outport  Port=2
  SAS_OK : Outport  Port=3
  SAS_MsgCount : Outport  Port=4
  SAS_CheckSum : Outport  Port=5
  Message_Checksum : Outport  Port=6
  wires:
  CAN1_Rx/1 -> [CAN1_Rx]
  [CAN1_Rx] -> Bus Selector/1
  Bus Selector/1 -> SAS_Angle/1  "<SAS_Angle>"
  Bus Selector/2 -> SAS_CAL/1  "<SAS_CAL>"
  Bus Selector/3 -> SAS_CheckSum/1  "<SAS_CheckSum>"
  Bus Selector/5 -> SAS_MsgCount/1, ChecksumCalculation/1(SAS_MsgCount)  "<SAS_MsgCount>"
  Bus Selector/4 -> SAS_OK/1  "<SAS_OK>"
  ChecksumCalculation/1(Message_Checksum) -> Message_Checksum/1
  [CAN1_Rx] -> ChecksumCalculation/2(CAN1_Rx)

== system hcu_main_ADASwEPS/dHAL_IN/dHAL_IN_EPAS/BO__926_EPAS2__8_EPAS ==
  CAN1_Rx : Inport
  Bus Selector : BusSelector  OutputSignals=EPAS2.Elect_PWR_Consumpt,EPAS2.EpasFailed,EPAS2.RSP_OK,EPAS2.R_SAS_Angle,EPAS2.Steering_Torque,EPAS2.Steering_Torque_V,EPAS2.SAS_CheckSum2,EPAS2.SAS_MsgCount2
  ChecksumCalculation : Subsystem  TreatAsAtomicUnit=on
  Elect_PWR_Consumpt : Outport
  EpasFailed : Outport  Port=2
  R_SAS_Angle : Outport  Port=3
  RSP_OK : Outport  Port=4
  SAS_MsgCount2 : Outport  Port=5
  Steering_Torque : Outport  Port=6
  Steering_Torque_V : Outport  Port=7
  SAS_CheckSum2 : Outport  Port=8
  Message_Checksum : Outport  Port=9
  wires:
  [CAN1_Rx] -> Bus Selector/1
  CAN1_Rx/1 -> [CAN1_Rx]
  Bus Selector/1 -> Elect_PWR_Consumpt/1  "<Elect_PWR_Consumpt>"
  Bus Selector/2 -> EpasFailed/1  "<EpasFailed>"
  Bus Selector/3 -> RSP_OK/1  "<RSP_OK>"
  Bus Selector/4 -> R_SAS_Angle/1  "<R_SAS_Angle>"
  Bus Selector/7 -> SAS_CheckSum2/1  "<SAS_CheckSum2>"
  Bus Selector/8 -> ChecksumCalculation/1(SAS_MsgCount), SAS_MsgCount2/1  "<SAS_MsgCount2>"
  Bus Selector/5 -> Steering_Torque/1  "<Steering_Torque>"
  Bus Selector/6 -> Steering_Torque_V/1  "<Steering_Torque_V>"
  ChecksumCalculation/1(Message_Checksum) -> Message_Checksum/1
  [CAN1_Rx] -> ChecksumCalculation/2(CAN1_Rx)

== system hcu_main_ADASwEPS/dHAL_IN/dHAL_IN_EPAS/CurStrAngReq_cvt ==
  value : Inport
  Add : Sum  Inputs=+-
  Data Type Conversion : DataTypeConversion  OutDataTypeStr=uint32  RndMeth=Nearest
  Divide : Product  Inputs=*/
  gain : Constant  Value=single(gain)  OutDataTypeStr=single
  offset : Constant  Value=single(offset)  OutDataTypeStr=single
  raw32 : Outport
  wires:
  value/1 -> Add/1
  offset/1 -> Add/2
  Divide/1 -> Data Type Conversion/1
  Add/1 -> Divide/1
  gain/1 -> Divide/2
  Data Type Conversion/1 -> raw32/1

== system hcu_main_ADASwEPS/dHAL_IN/dHAL_IN_EPAS/CurStrTqReq_cvt ==
  value : Inport
  Add : Sum  Inputs=+-
  Data Type Conversion : DataTypeConversion  OutDataTypeStr=uint32  RndMeth=Nearest
  Divide : Product  Inputs=*/
  gain : Constant  Value=single(gain)  OutDataTypeStr=single
  offset : Constant  Value=single(offset)  OutDataTypeStr=single
  raw32 : Outport
  wires:
  Data Type Conversion/1 -> raw32/1
  gain/1 -> Divide/2
  Add/1 -> Divide/1
  Divide/1 -> Data Type Conversion/1
  offset/1 -> Add/2
  value/1 -> Add/1

== system hcu_main_ADASwEPS/dHAL_IN/dHAL_IN_EPAS/EPSBattVolt_cvt ==
  value : Inport
  Add : Sum  Inputs=+-
  Data Type Conversion : DataTypeConversion  OutDataTypeStr=uint32  RndMeth=Nearest
  Divide : Product  Inputs=*/
  gain : Constant  Value=single(gain)  OutDataTypeStr=single
  offset : Constant  Value=single(offset)  OutDataTypeStr=single
  raw32 : Outport
  wires:
  value/1 -> Add/1
  offset/1 -> Add/2
  Divide/1 -> Data Type Conversion/1
  Add/1 -> Divide/1
  gain/1 -> Divide/2
  Data Type Conversion/1 -> raw32/1

== system hcu_main_ADASwEPS/dHAL_IN/dHAL_IN_EPAS/R_SAS_Angle_cvt ==
  value : Inport
  Add : Sum  Inputs=+-
  Data Type Conversion : DataTypeConversion  OutDataTypeStr=uint32  RndMeth=Nearest
  Divide : Product  Inputs=*/
  gain : Constant  Value=single(gain)  OutDataTypeStr=single
  offset : Constant  Value=single(offset)  OutDataTypeStr=single
  raw32 : Outport
  wires:
  value/1 -> Add/1
  offset/1 -> Add/2
  Divide/1 -> Data Type Conversion/1
  Add/1 -> Divide/1
  gain/1 -> Divide/2
  Data Type Conversion/1 -> raw32/1

== system hcu_main_ADASwEPS/dHAL_IN/dHAL_IN_EPAS/SAS_Angle_cvt ==
  value : Inport
  Add : Sum  Inputs=+-
  Data Type Conversion : DataTypeConversion  OutDataTypeStr=uint32  RndMeth=Nearest
  Divide : Product  Inputs=*/
  gain : Constant  Value=single(gain)  OutDataTypeStr=single
  offset : Constant  Value=single(offset)  OutDataTypeStr=single
  raw32 : Outport
  wires:
  Data Type Conversion/1 -> raw32/1
  gain/1 -> Divide/2
  Add/1 -> Divide/1
  Divide/1 -> Data Type Conversion/1
  offset/1 -> Add/2
  value/1 -> Add/1

== system hcu_main_ADASwEPS/dHAL_IN/dHAL_IN_METER/BO__1104_Meter1__8_Meter ==
  CAN1_Rx : Inport
  Bus Selector : BusSelector  OutputSignals=Meter1.LowBrakeFluid_Sta,Meter1.ODOMETER,Meter1.ParkBrake,Meter1.SeatBelt
  LowBrakeFluid_Sta : Outport
  ODOMETER : Outport  Port=2
  ParkBrake : Outport  Port=3
  SeatBelt : Outport  Port=4
  wires:
  CAN1_Rx/1 -> [CAN1_Rx]
  [CAN1_Rx] -> Bus Selector/1
  Bus Selector/4 -> SeatBelt/1  "<SeatBelt>"
  Bus Selector/3 -> ParkBrake/1  "<ParkBrake>"
  Bus Selector/2 -> ODOMETER/1  "<ODOMETER>"
  Bus Selector/1 -> LowBrakeFluid_Sta/1  "<LowBrakeFluid_Sta>"

== system hcu_main_ADASwEPS/dHAL_IN/dHAL_IN_METER/BO__1306_Meter3__8_Meter ==
  CAN1_Rx : Inport
  Bus Selector : BusSelector  OutputSignals=Meter3.Meter_Ind_VehSpeed
  Meter_Ind_VehSpeed : Outport
  wires:
  [CAN1_Rx] -> Bus Selector/1
  CAN1_Rx/1 -> [CAN1_Rx]
  Bus Selector/1 -> Meter_Ind_VehSpeed/1  "<Meter_Ind_VehSpeed>"

== system hcu_main_ADASwEPS/dHAL_IN/dHAL_IN_METER/Meter_Ind_VehSpeed_cvt ==
  value : Inport
  Add : Sum  Inputs=+-
  Data Type Conversion : DataTypeConversion  OutDataTypeStr=uint32  RndMeth=Nearest
  Divide : Product  Inputs=*/
  gain : Constant  Value=single(gain)  OutDataTypeStr=single
  offset : Constant  Value=single(offset)  OutDataTypeStr=single
  raw32 : Outport
  wires:
  Data Type Conversion/1 -> raw32/1
  gain/1 -> Divide/2
  Add/1 -> Divide/1
  Divide/1 -> Data Type Conversion/1
  offset/1 -> Add/2
  value/1 -> Add/1

== system hcu_main_ADASwEPS/dHAL_IN/dHAL_IN_METER/ODOMETER_cvt ==
  value : Inport
  Add : Sum  Inputs=+-
  Data Type Conversion : DataTypeConversion  OutDataTypeStr=uint32  RndMeth=Nearest
  Divide : Product  Inputs=*/
  gain : Constant  Value=single(gain)  OutDataTypeStr=single
  offset : Constant  Value=single(offset)  OutDataTypeStr=single
  raw32 : Outport
  wires:
  value/1 -> Add/1
  offset/1 -> Add/2
  Divide/1 -> Data Type Conversion/1
  Add/1 -> Divide/1
  gain/1 -> Divide/2
  Data Type Conversion/1 -> raw32/1

== system hcu_main_ADASwEPS/dHAL_IN/dHAL_IN_TCM/BO__832_TCM1__8_TCM ==
  CAN1_Rx : Inport
  Bus Selector : BusSelector  OutputSignals=TCM1.CAN_ETCU_STATE,TCM1.CAN_GEAR_SEL_ETCU,TCM1.CAN_GEAR_STATE_NOW,TCM1.CAN_GEAR_STA_NOW_V,TCM1.CAN_N_TM,TCM1.LV_CAN_N_TM_ERR,TCM1.CAN_SWI_CC_ETCU,TCM1.CAN_ETCU_OBD,TCM1.CAN_WTR,TCM1.CAN_PWR
  CAN_ETCU_STATE : Outport
  CAN_GEAR_SEL_ETCU : Outport  Port=2
  CAN_GEAR_STATE_NOW : Outport  Port=3
  CAN_GEAR_STA_NOW_V : Outport  Port=4
  CAN_N_TM : Outport  Port=5
  LV_CAN_N_TM_ERR : Outport  Port=6
  CAN_SWI_CC_ETCU : Outport  Port=7
  CAN_ETCU_OBD : Outport  Port=8
  CAN_WTR : Outport  Port=9
  CAN_PWR : Outport  Port=10
  wires:
  CAN1_Rx/1 -> [CAN1_Rx]
  [CAN1_Rx] -> Bus Selector/1
  Bus Selector/1 -> CAN_ETCU_STATE/1  "<CAN_ETCU_STATE>"
  Bus Selector/2 -> CAN_GEAR_SEL_ETCU/1  "<CAN_GEAR_SEL_ETCU>"
  Bus Selector/3 -> CAN_GEAR_STATE_NOW/1  "<CAN_GEAR_STATE_NOW>"
  Bus Selector/4 -> CAN_GEAR_STA_NOW_V/1  "<CAN_GEAR_STA_NOW_V>"
  Bus Selector/5 -> CAN_N_TM/1  "<CAN_N_TM>"
  Bus Selector/6 -> LV_CAN_N_TM_ERR/1  "<LV_CAN_N_TM_ERR>"
  Bus Selector/7 -> CAN_SWI_CC_ETCU/1  "<CAN_SWI_CC_ETCU>"
  Bus Selector/8 -> CAN_ETCU_OBD/1  "<CAN_ETCU_OBD>"
  Bus Selector/9 -> CAN_WTR/1  "<CAN_WTR>"
  Bus Selector/10 -> CAN_PWR/1  "<CAN_PWR>"

== system hcu_main_ADASwEPS/dHAL_IN/dHAL_IN_TCM/BO__842_TCM2__8_TCM ==
  CAN1_Rx : Inport
  Bus Selector : BusSelector  OutputSignals=TCM2.DR_MODE_IND
  DR_MODE_IND : Outport
  wires:
  [CAN1_Rx] -> Bus Selector/1
  CAN1_Rx/1 -> [CAN1_Rx]
  Bus Selector/1 -> DR_MODE_IND/1  "<DR_MODE_IND>"
